simulink model "HT1_model"  (R2023a)
settings: Solver=VariableStepAuto  StartTime=0.0  StopTime=10.0  RelTol=1e-3
values from neighbouring files (symbols this model uses):
  k1 = 20    [HT1.m]
  k2 = 45    [HT1.m]
  T = 7    [HT1.m]
  T1 = 0.025    [HT1.m]
settings Model: Creator=User  LastModifiedBy=User

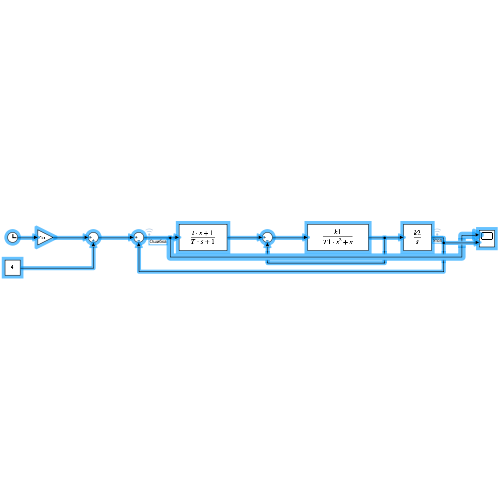
[thumbnail: Simulink's stored preview of the top-level diagram]
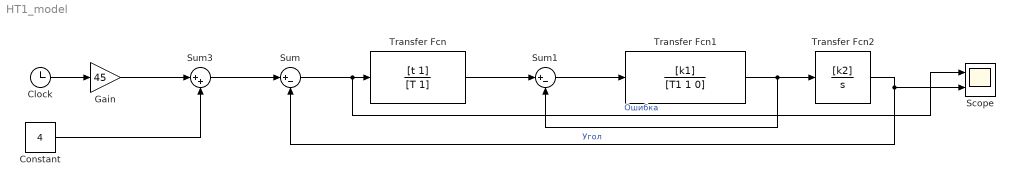
== system HT1_model ==
  Clock : Clock
  Constant : Constant  Value=4
  Gain : Gain  Gain=45
  Scope : Scope  NumInputPorts=2
  Sum : Sum  Inputs=|+-
  Sum1 : Sum  Inputs=|+-
  Sum3 : Sum  Inputs=|++
  Transfer Fcn : TransferFcn  Numerator=[t 1]  Denominator=[T 1]
  Transfer Fcn1 : TransferFcn  Numerator=[k1]  Denominator=[T1 1 0]
  Transfer Fcn2 : TransferFcn  Numerator=[k2]  Denominator=[1 0]
  wires:
  Gain/1 -> Sum3/1
  Sum1/1 -> Transfer Fcn1/1
  Sum3/1 -> Sum/1
  Constant/1 -> Sum3/2
  Transfer Fcn2/1 -> Scope/2, Sum/2  "Угол"
  Clock/1 -> Gain/1
  Transfer Fcn/1 -> Sum1/1
  Transfer Fcn1/1 -> Sum1/2, Transfer Fcn2/1
  Sum/1 -> Scope/1, Transfer Fcn/1  "Ошибка"
